simulink model "supertwistingControl"  (R2018a)
settings: Solver=ode1  StartTime=0.0  StopTime=10  FixedStep=0.001  RelTol=1e-3
settings Model: Creator=27154  LastModifiedBy=27154
settings SolverCC: ZeroCrossAlgorithm=Adaptive
settings DebuggingCC: MaxConsecutiveZCsMsg=none

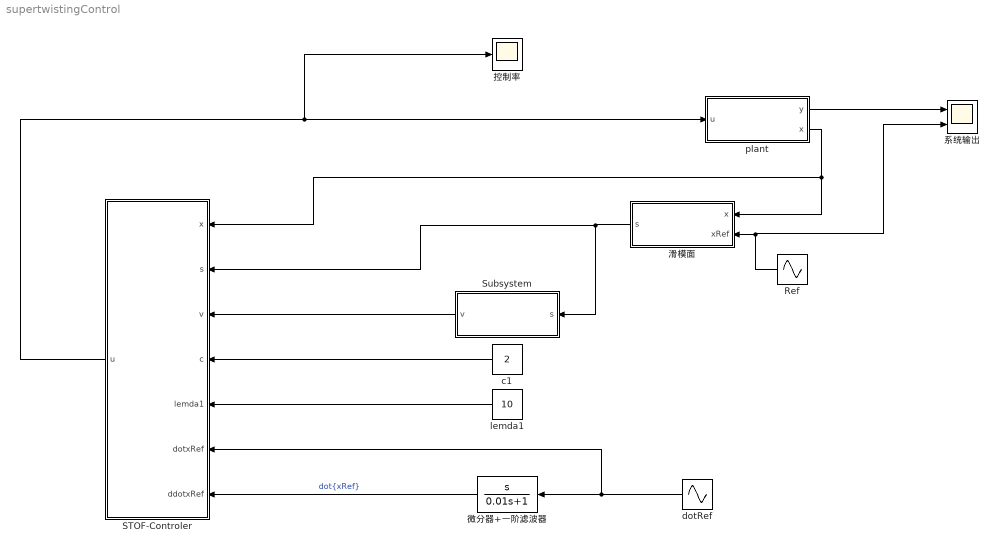
== system supertwistingControl ==
  Ref : Sin  SampleTime=0
  STOF-Controler : MATLAB Function  TreatAsAtomicUnit=on
  Subsystem : Subsystem  mask{lemda2=100}
      mask prompts: lemda2 "参数：lemda2"
  c1 : Constant  Value=2
  dotRef : Sin  Phase=pi/2  SampleTime=0
  lemda1 : Constant  Value=10
  plant : Subsystem  mask{A=[0 1; 0 -8.4344], b=[0; 458.46], c=[1 0], x0=[0; 0]}
      mask prompts: A "系统参数：A"; b "系统参数：b"; c "系统参数：c"; x0 "初始状态：x"
  微分器+一阶滤波器 : TransferFcn  Numerator=[1 0]  Denominator=[0.01 1]
  控制率 : Scope
  滑模面 : Subsystem  mask{c=2}
      mask prompts: c "参数：c"
  系统输出 : Scope  NumInputPorts=2
  wires:
  STOF-Controler/1(u) -> plant/1(u), 控制率/1
  plant/2("x ") -> STOF-Controler/1(x), 滑模面/1(x)
  Ref/1 -> 系统输出/2, 滑模面/2(xRef)
  滑模面/1(s) -> STOF-Controler/2(s), Subsystem/1(s)
  Subsystem/1(v) -> STOF-Controler/3(v)
  c1/1 -> STOF-Controler/4(c)
  lemda1/1 -> STOF-Controler/5(lemda1)
  微分器+一阶滤波器/1 -> STOF-Controler/7(ddotxRef)  "dot{xRef}"
  dotRef/1 -> STOF-Controler/6(dotxRef), 微分器+一阶滤波器/1
  plant/1(y) -> 系统输出/1

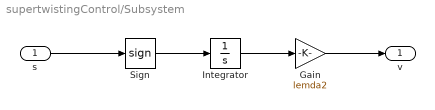
== system supertwistingControl/Subsystem ==
  s : Inport
  Gain : Gain  Gain=lemda2
  Integrator : Integrator
  Sign : Signum
  v : Outport
  wires:
  s/1 -> Sign/1
  Integrator/1 -> Gain/1
  Sign/1 -> Integrator/1
  Gain/1 -> v/1

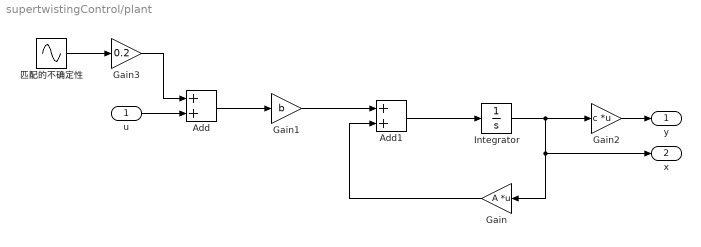
== system supertwistingControl/plant ==
  u : Inport
  Add : Sum
  Add1 : Sum
  Gain : Gain  Gain=A  Multiplication=Matrix(K*u) (u vector)
  Gain1 : Gain  Gain=b
  Gain2 : Gain  Gain=c  Multiplication=Matrix(K*u) (u vector)
  Gain3 : Gain  Gain=0.2
  Integrator : Integrator  InitialCondition=x0
  匹配的不确定性 : Sin  SampleTime=0
  y : Outport
  "x " : Outport  Port=2
  wires:
  Integrator/1 -> "x "/1, Gain/1, Gain2/1
  u/1 -> Add/2
  Add/1 -> Gain1/1
  Gain1/1 -> Add1/1
  Add1/1 -> Integrator/1
  Gain/1 -> Add1/2
  Gain2/1 -> y/1
  匹配的不确定性/1 -> Gain3/1
  Gain3/1 -> Add/1

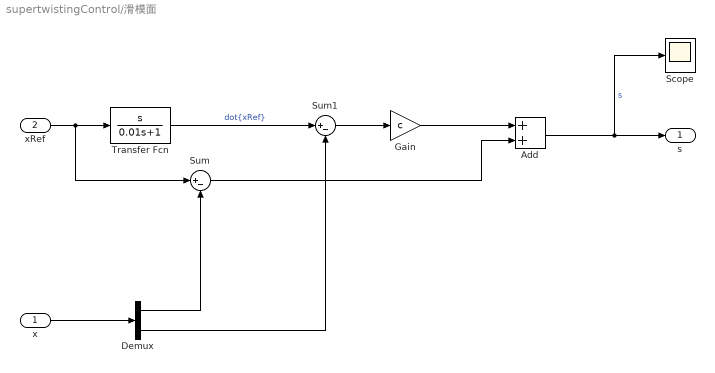
== system supertwistingControl/滑模面 ==
  x : Inport
  xRef : Inport  Port=2
  Add : Sum
  Demux : Demux  Outputs=2
  Gain : Gain  Gain=c
  Scope : Scope
  Sum : Sum  Inputs=|+-
  Sum1 : Sum  Inputs=|+-
  Transfer Fcn : TransferFcn  Numerator=[1 0]  Denominator=[0.01 1]
  s : Outport
  wires:
  xRef/1 -> Sum/1, Transfer Fcn/1
  x/1 -> Demux/1
  Demux/1 -> Sum/2
  Transfer Fcn/1 -> Sum1/1  "dot{xRef}"
  Demux/2 -> Sum1/2
  Sum1/1 -> Gain/1
  Sum/1 -> Add/2
  Gain/1 -> Add/1
  Add/1 -> Scope/1, s/1  "s"

== matlab function supertwistingControl/STOF-Controler ==
  data: x input; s input; v input; c input; lemda1 input; dotxRef input; u output; ddotxRef input
function u = fcn(x, s, v, c, lemda1, dotxRef, ddotxRef)

x2 = x(2);

%u = -c1 * x2 - x3 - k2 * abs(e1)^(1/3) * sign(e1) - lemda1 * abs(s)^(1/2) * sign(s) + v;

u = 1/458.46 * (-c * x2 + 8.4344 * x2 + c * dotxRef + ddotxRef + lemda1 * abs(s)^(1/2) * sign(s) + v);
